simulink model "model_dynamik_w"  (R2023b)
settings: Solver=VariableStepAuto  StartTime=0.0  StopTime=10.0  RelTol=1e-3
values from neighbouring files (symbols this model uses):
  tau = 1    [parametry.m]
settings Model: Creator=Jakub  LastModifiedBy=Jakub

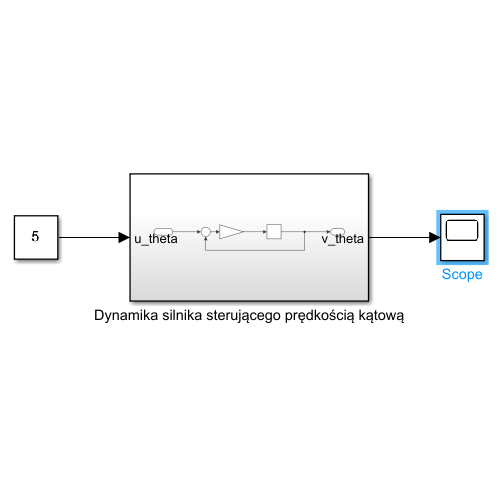
[thumbnail: Simulink's stored preview of the top-level diagram]
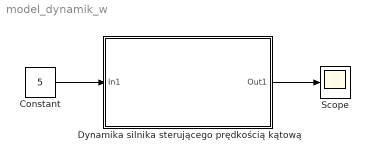
== system model_dynamik_w ==
  Constant : Constant  Value=5
  Dynamika silnika sterującego prędkością kątową : Subsystem
  Scope : Scope
  wires:
  Constant/1 -> Dynamika silnika sterującego prędkością kątową/1(In1)
  Dynamika silnika sterującego prędkością kątową/1(Out1) -> Scope/1

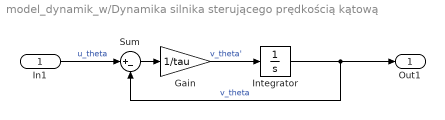
== system model_dynamik_w/Dynamika silnika sterującego prędkością kątową ==
  In1 : Inport
  Gain : Gain  Gain=1/tau
  Integrator : Integrator
  Sum : Sum  Inputs=|+-
  Out1 : Outport
  wires:
  Integrator/1 -> Out1/1, Sum/2  "v_theta"
  Gain/1 -> Integrator/1  "v_theta'"
  In1/1 -> Sum/1  "u_theta"
  Sum/1 -> Gain/1
